simulink model "nms_model"  (Simulink 7.5)
settings: Solver=ode15s  StartTime=0.0  StopTime=60  FixedStep=1e-3  MaxStep=ts_max  RelTol=1e-3  AbsTol=1e-4
InitFcn:
  | nms_model_MechInit
  | nms_model_ControlInit
values from neighbouring files (symbols this model uses):
  c = 0.05    [muscleParams.m]    (also in nms_model_MechInit.m)
  c_jointstop = 0.3 / (pi/180)    (= 17.1887338539)    [muscleParams.m]    (also in nms_model_MechInit.m)
  D12_F = 0.16    [nms_model_MechInit.m]
  D12_S = L_S    (= 0.5)    [nms_model_MechInit.m]
  D12_T = L_T    (= 0.5)    [nms_model_MechInit.m]
  D13_F = 0.20    (= 0.2)    [nms_model_MechInit.m]
  D1G_F = 0.14    [nms_model_MechInit.m]
  D1G_HAT = 0.35    [nms_model_MechInit.m]
  D1G_S = 0.3    [nms_model_MechInit.m]
  D1G_T = 0.3    [nms_model_MechInit.m]
  DeltaThRef = 5e-3    (= 0.005)    [nms_model_MechInit.m]
  eref = 0.04    [muscleParams.m]    (also in nms_model_MechInit.m)
  FmaxGAS = 1500    [nms_model_MechInit.m]
  FmaxGLU = 1500    [nms_model_MechInit.m]
  FmaxHAM = 3000    [nms_model_MechInit.m]
  FmaxHFL = 2000    [nms_model_MechInit.m]
  FmaxSOL = 4000    [nms_model_MechInit.m]
  FmaxTA = 800    [nms_model_MechInit.m]
  FmaxVAS = 300    [muscleParams.m]    (also in nms_model_MechInit.m = 6000)
  GainDeltaTheta = 2 /100*180/pi    (= 1.14591559026)    [nms_model_ControlInit.m]
  GainGAS = 1.1/FmaxGAS    [nms_model_ControlInit.m]
  GainGLU = 0.5/FmaxGLU    [nms_model_ControlInit.m]
  GainHAM = 0.65/FmaxHAM    [nms_model_ControlInit.m]
  GainHAMHFL = 4    [nms_model_ControlInit.m]
  GainHFL = 0.5    [nms_model_ControlInit.m]
  GainKneOverExt = 2    [nms_model_ControlInit.m]
  GainSOL = 1.2/FmaxSOL    [nms_model_ControlInit.m]
  GainSOLTA = 0.4/FmaxSOL    [nms_model_ControlInit.m]
  GainTA = 1.1    [nms_model_ControlInit.m]
  GainVAS = 1.2/FmaxVAS    [nms_model_ControlInit.m]
  In_F = 0.005    [nms_model_MechInit.m]
  In_HAT = 3    [nms_model_MechInit.m]
  In_S = 0.05    [nms_model_MechInit.m]
  In_T = 0.15    [nms_model_MechInit.m]
  K = 5    [muscleParams.m]    (also in nms_model_MechInit.m)
  k_gx = (2*(m_F+m_S+m_T)+m_HAT)*g/0.1    (= 7848)    [nms_model_MechInit.m]
  k_gy = (2*(m_F+m_S+m_T)+m_HAT)*g/0.01    (= 78480)    [nms_model_MechInit.m]
  k_pressure = m_HAT * 9.81 / DeltaThRef    (= 104967)    [nms_model_MechInit.m]
  K_swing = 0.25    [nms_model_ControlInit.m]
  KneePh23Offset = 170*pi/180    (= 2.96705972839)    [nms_model_ControlInit.m]
  LceOffsetHAM = 0.85    [nms_model_ControlInit.m]
  LceOffsetHFL = 0.65    [nms_model_ControlInit.m]
  LceOffsetTA = 1-0.5*w    [nms_model_ControlInit.m]
  LongDelay = 0.020    (= 0.02)    [nms_model_ControlInit.m]
  loptGAS = 0.05    [nms_model_MechInit.m]
  loptGLU = 0.11    [nms_model_MechInit.m]
  loptHAM = 0.10    (= 0.1)    [nms_model_MechInit.m]
  loptHFL = 0.11    [nms_model_MechInit.m]
  loptSOL = 0.04    [nms_model_MechInit.m]
  loptTA = 0.06    [nms_model_MechInit.m]
  loptVAS = 0.13    [muscleParams.m]    (also in nms_model_MechInit.m = 0.08)
  lslackGAS = 0.40    (= 0.4)    [nms_model_MechInit.m]
  lslackGLU = 0.13    [nms_model_MechInit.m]
  lslackHAM = 0.31    [nms_model_MechInit.m]
  lslackHFL = 0.10    (= 0.1)    [nms_model_MechInit.m]
  lslackSOL = 0.26    [nms_model_MechInit.m]
  lslackTA = 0.24    [nms_model_MechInit.m]
  lslackVAS = 0.23    [muscleParams.m]    (also in nms_model_MechInit.m)
  m_F = 1.25    [nms_model_MechInit.m]
  m_HAT = 53.5    [nms_model_MechInit.m]
  m_S = 3.5    [nms_model_MechInit.m]
  m_T = 8.5    [nms_model_MechInit.m]
  MidDelay = 0.010    (= 0.01)    [nms_model_ControlInit.m]
  mu_slide = 0.8    [nms_model_MechInit.m]
  mu_stick = 0.9    [nms_model_MechInit.m]
  N = 1.5    [muscleParams.m]    (also in nms_model_MechInit.m)
  phi12_LowLimit = 70*pi/180    (= 1.2217304764)    [nms_model_MechInit.m]
  phi12_UpLimit = 180*pi/180    (= 3.14159265359)    [muscleParams.m]    (also in nms_model_MechInit.m = 2.26892802759)
  phi23_UpLimit = 159*pi/180    (= 2.77507351067)    [muscleParams.m]    (also in nms_model_MechInit.m = 3.05432619099)
  phi34_UpLimit = 230*pi/180    (= 4.01425727959)    [nms_model_MechInit.m]
  phimaxGASa = 110*pi/180    (= 1.91986217719)    [nms_model_MechInit.m]
  phimaxGASk = 140*pi/180    (= 2.44346095279)    [nms_model_MechInit.m]
  phimaxHAMk = 180*pi/180    (= 3.14159265359)    [nms_model_MechInit.m]
  phimaxSOL = 110*pi/180    (= 1.91986217719)    [nms_model_MechInit.m]
  phimaxTA = 80*pi/180    (= 1.3962634016)    [nms_model_MechInit.m]
  phimaxVAS = 90*pi/180    (= 1.57079632679)    [muscleParams.m]    (also in nms_model_MechInit.m = 2.87979326579)
  phirefGASa = 80*pi/180    (= 1.3962634016)    [nms_model_MechInit.m]
  phirefGASk = 165*pi/180    (= 2.87979326579)    [nms_model_MechInit.m]
  phirefGLU = 150*pi/180    (= 2.61799387799)    [nms_model_MechInit.m]
  phirefHAMh = 155*pi/180    (= 2.70526034059)    [nms_model_MechInit.m]
  phirefHAMk = 180*pi/180    (= 3.14159265359)    [nms_model_MechInit.m]
  phirefHFL = 180*pi/180    (= 3.14159265359)    [nms_model_MechInit.m]
  phirefSOL = 80*pi/180    (= 1.3962634016)    [nms_model_MechInit.m]
  phirefTA = 110*pi/180    (= 1.91986217719)    [nms_model_MechInit.m]
  phirefVAS = 60*pi/180    (= 1.0471975512)    [muscleParams.m]    (also in nms_model_MechInit.m = 2.18166156499)
  PosGainGG = 1/(30*pi/180)    (= 1.9098593171)    [nms_model_ControlInit.m]
  PreStimGAS = 0.01    [nms_model_ControlInit.m]
  PreStimGG = 0.05    [nms_model_ControlInit.m]
  PreStimGLU = 0.01    [nms_model_ControlInit.m]
  PreStimHAM = 0.01    [nms_model_ControlInit.m]
  PreStimHFL = 0.01    [nms_model_ControlInit.m]
  PreStimSOL = 0.01    [nms_model_ControlInit.m]
  PreStimTA = 0.01    [nms_model_ControlInit.m]
  PreStimVAS = 0.08    [nms_model_ControlInit.m]
  rGASa = 0.05    [nms_model_MechInit.m]
  rGASk = 0.05    [nms_model_MechInit.m]
  rGLU = 0.10    (= 0.1)    [nms_model_MechInit.m]
  rHAMh = 0.08    [nms_model_MechInit.m]
  rHAMk = 0.05    [nms_model_MechInit.m]
  rHFL = 0.10    (= 0.1)    [nms_model_MechInit.m]
  rhoGASa = 0.7    [nms_model_MechInit.m]
  rhoGASk = 0.7    [nms_model_MechInit.m]
  rhoGLU = 0.5    [nms_model_MechInit.m]
  rhoHAMh = 0.7    [nms_model_MechInit.m]
  rhoHAMk = 0.7    [nms_model_MechInit.m]
  rhoHFL = 0.5    [nms_model_MechInit.m]
  rhoSOL = 0.5    [nms_model_MechInit.m]
  rhoTA = 0.7    [nms_model_MechInit.m]
  rhoVAS = 3    [muscleParams.m]    (also in nms_model_MechInit.m = 0.7)
  rSOL = 0.05    [nms_model_MechInit.m]
  rTA = 0.04    [nms_model_MechInit.m]
  rVAS = 0.03    [muscleParams.m]    (also in nms_model_MechInit.m = 0.06)
  s = orProblemSendCommand(['LoadIKFastSolver robot Translation3D'],probid)    [init.m]
  ShortDelay = 0.005    [nms_model_ControlInit.m]
  SpeedGainGG = 0.2    [nms_model_ControlInit.m]
  tau = 0.01    [muscleParams.m]    (also in nms_model_MechInit.m)
  Theta0 = 6*pi/180    (= 0.10471975512)    [nms_model_ControlInit.m]
  ThPos = 4/5    (= 0.8)    [nms_model_MechInit.m]
  v_gx_max = 0.03    [nms_model_MechInit.m]
  v_gy_max = 0.03    [nms_model_MechInit.m]
  ... (+11 more)
undefined symbols (not defined in the file or in its folder): sgn
libraries: mblibv1 x60, simulink x22, simulink_extras x20
(part 2 of 9)

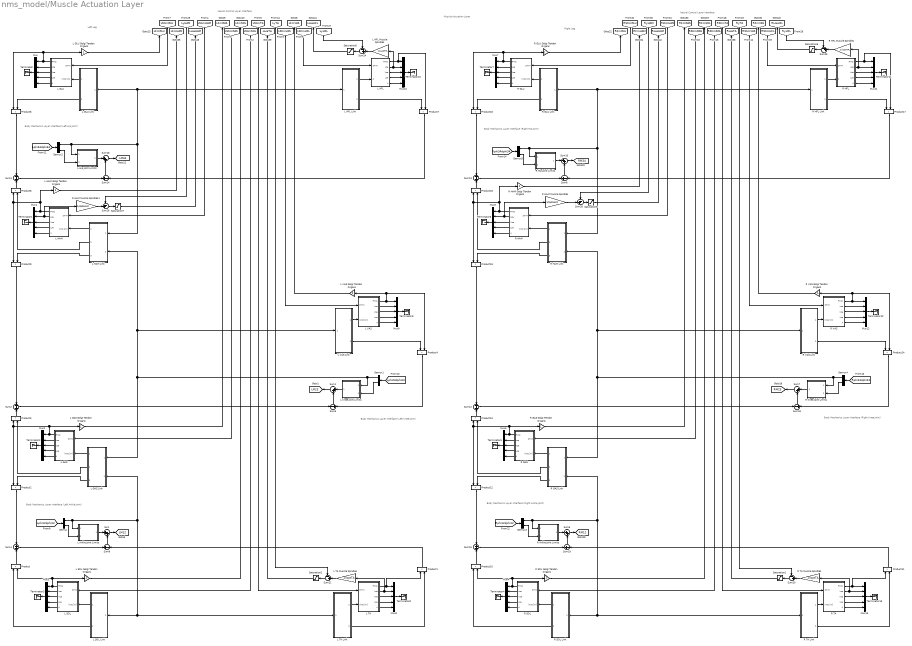
== system nms_model/Muscle Actuation Layer ==
  note: Left Leg
  note: Neural Control Layer Interface
  note: Body Mechanics Layer
      | Interface (Left Hip Joint)
  note: Body Mechanics Layer
      | Interface (Left Knee Joint)
  note: Body Mechanics Layer
      | Interface (Left Ankle Joint)
  note: Neural Control Layer Interface
  note: Body Mechanics Layer
      | Interface (Right Hip Joint)
  note: Body Mechanics Layer
      | Interface (Right Knee Joint)
  note: Body Mechanics Layer
      | Interface (Right Ankle Joint)
  note: Right Leg
  note: Muscle Actuation Layer
  Demux{,1..5} (6 alike) : Demux  Outputs=2
  L Ankle Joint Limits : Subsystem
  L GAS : Subsystem
  L GAS Golgi Tendon Organs : Gain  ParameterDataType=sfix(16)  ParameterScaling=2^0  OutDataType=sfix(16)  OutScaling=2^0
  L GAS Link : Subsystem
  L GLU : Subsystem
  L GLU Golgi Tendon Organs : Gain  ParameterDataType=sfix(16)  ParameterScaling=2^0  OutDataType=sfix(16)  OutScaling=2^0
  L GLU Link : Subsystem
  L HAM : Subsystem
  L HAM Golgi Tendon Organs : Gain  ParameterDataType=sfix(16)  ParameterScaling=2^0  OutDataType=sfix(16)  OutScaling=2^0
  L HAM Link : Subsystem
  L HFL : Subsystem
  L HFL Muscle Spindles : Gain  Gain=1/loptHFL  ParameterDataType=sfix(16)  ParameterScaling=2^0  OutDataType=sfix(16)  OutScaling=2^0
  L HFL Link : Subsystem
  L Hip Joint Limits : Subsystem
  L Knee Joint Limits : Subsystem
  L SOL : Subsystem
  L SOL Golgi Tendon Organs : Gain  ParameterDataType=sfix(16)  ParameterScaling=2^0  OutDataType=sfix(16)  OutScaling=2^0
  L SOL Link : Subsystem
  L TA : Subsystem
  L TA Muscle Spindles : Gain  Gain=1/loptTA  ParameterDataType=sfix(16)  ParameterScaling=2^0  OutDataType=sfix(16)  OutScaling=2^0
  L TA Link : Subsystem
  L VAS : Subsystem
  L VAS Golgi Tendon Organs : Gain  ParameterDataType=sfix(16)  ParameterScaling=2^0  OutDataType=sfix(16)  OutScaling=2^0
  L VAS Link : Subsystem
  Mux{,1..13} (14 alike) : Mux  Inputs=5
  Product{,1..4,6..14,16..19} (18 alike) : Product  OutDataType=sfix(16)  OutScaling=2^0  RndMeth=Zero
  R Ankle Joint Limits : Subsystem
  R GAS : Subsystem
  R GAS Golgi Tendon Organs : Gain  ParameterDataType=sfix(16)  ParameterScaling=2^0  OutDataType=sfix(16)  OutScaling=2^0
  R GAS Link : Subsystem
  R GLU : Subsystem
  R GLU Golgi Tendon Organs : Gain  ParameterDataType=sfix(16)  ParameterScaling=2^0  OutDataType=sfix(16)  OutScaling=2^0
  R GLU Link : Subsystem
  R HAM : Subsystem
  R HAM Golgi Tendon Organs : Gain  ParameterDataType=sfix(16)  ParameterScaling=2^0  OutDataType=sfix(16)  OutScaling=2^0
  R HAM Muscle Spindles : Gain  Gain=1/loptHAM  ParameterDataType=sfix(16)  ParameterScaling=2^0  OutDataType=sfix(16)  OutScaling=2^0
  R HAM Muscle Spindles1 : Gain  Gain=1/loptHAM  ParameterDataType=sfix(16)  ParameterScaling=2^0  OutDataType=sfix(16)  OutScaling=2^0
  R HAM Link : Subsystem
  R HFL : Subsystem
  R HFL Muscle Spindles : Gain  Gain=1/loptHFL  ParameterDataType=sfix(16)  ParameterScaling=2^0  OutDataType=sfix(16)  OutScaling=2^0
  R HFL Link : Subsystem
  R Hip Joint Limits : Subsystem
  R Knee Joint Limits : Subsystem
  R SOL : Subsystem
  R SOL Golgi Tendon Organs : Gain  ParameterDataType=sfix(16)  ParameterScaling=2^0  OutDataType=sfix(16)  OutScaling=2^0
  R SOL Link : Subsystem
  R TA : Subsystem
  R TA Muscle Spindles : Gain  Gain=1/loptTA  ParameterDataType=sfix(16)  ParameterScaling=2^0  OutDataType=sfix(16)  OutScaling=2^0
  R TA Link : Subsystem
  R VAS : Subsystem
  R VAS Golgi Tendon Organs : Gain  ParameterDataType=sfix(16)  ParameterScaling=2^0  OutDataType=sfix(16)  OutScaling=2^0
  R VAS Link : Subsystem
  Saturation{1..2,5..7,9} (6 alike) : Saturate  UpperLimit=inf  LowerLimit=0  ZeroCross=off
  Sum{,1,6..7,10,16} (6 alike) : Sum  Inputs=|++  OutDataType=sfix(16)  OutScaling=2^0
  Sum{2..4,12..13,15} (6 alike) : Sum  OutDataType=sfix(16)  OutScaling=2^0
  Sum{8..9,14,19} (4 alike) : Sum  Inputs=+-  OutDataType=sfix(16)  OutScaling=2^0
  Sum18 : Sum  Inputs=-+  OutDataType=sfix(16)  OutScaling=2^0
  Sum{20..21,24..26,28} (6 alike) : Sum  Inputs=-+|  OutDataType=sfix(16)  OutScaling=2^0  SaturateOnIntegerOverflow=on  InputSameDT=on  OutDataTypeStr=Inherit: Same as first input
  Sum5 : Sum  Inputs=-+  OutDataType=sfix(16)  OutScaling=2^0
  Terminator{,1..13} (14 alike) : Terminator
  tag scope: LFmGAS=global, LFmGLU=global, LFmHAM=global, LFmSOL=global, LFmVAS=global, LLceHAM=global, LLceHFL=global, LLceTA=global, LM12=global, LM23=global, LM34=global, RFmGAS=global, RFmGLU=global, RFmHAM=global, RFmSOL=global, RFmVAS=global, RLceHAM=global, RLceHFL=global, RLceTA=global, RM12=global, RM23=global, RM34=global
  wires:
  Demux1/1 -> L Knee Joint Limits/1(phi [rad]), L VAS Link/1(phi23 [rad]), L HAM Link/2(phi23 [rad]), L GAS Link/1(phi23 [rad])
  L SOL/1(Fmtc) -> Product/2, L SOL Golgi Tendon Organs/1, Mux3/1
  L TA/1(Fmtc) -> Product1/1, Mux8/1
  L TA/2(Lce) -> L TA Muscle Spindles/1, Mux8/2
  L TA/5(A) -> Mux8/5
  L GAS/1(Fmtc) -> Product2/1, Product3/1, L GAS Golgi Tendon Organs/1, Mux2/1
  Demux/1 -> L SOL Link/1(phi12 [rad]), L TA Link/1(phi12 [rad]), L GAS Link/2(phi12 [rad]), L Ankle Joint Limits/1(phi [rad])
  [LStimTA] -> L TA/1(STIM)
  [LStimSOL] -> L SOL/1(STIM)
  [LStimHAM] -> L HAM/1(STIM)
  L HAM/1(Fmtc) -> Product9/1, Product8/1, L HAM Golgi Tendon Organs/1, Mux1/1
  L HAM/2(Lce) -> R HAM Muscle Spindles1/1, Mux1/2
  L HFL/1(Fmtc) -> Product7/2, Mux10/1
  L HFL/2(Lce) -> L HFL Muscle Spindles/1, Mux10/2
  [LStimHFL] -> L HFL/1(STIM)
  L GLU/1(Fmtc) -> Product6/1, L GLU Golgi Tendon Organs/1, Mux/1
  [LStimGLU] -> L GLU/1(STIM)
  Sum16/1 -> [LM34]
  Demux/2 -> L Ankle Joint Limits/2(dphi [rad/s])
  Sum9/1 -> Sum/2
  Demux1/2 -> L Knee Joint Limits/2(dphi [rad/s])
  L SOL Link/1(lmtc [m]) -> L SOL/2(lmtc [m])
  L TA Link/1(lmtc [m]) -> L TA/2(lmtc [m])
  L GAS Link/3(lever12 [m]) -> Product2/2
  L GAS Link/2(lever23 [m]) -> Product3/2
  [LStimGAS] -> L GAS/1(STIM)
  L GAS Link/1(lmtu [m]) -> L GAS/2(lmtc [m])
  L VAS Link/1(lmtu [m]) -> L VAS/2(lmtc [m])
  Product4/1 -> Sum5/2
  L HAM Link/1(lmtu [m]) -> L HAM/2(lmtc [m])
  L HAM Link/2(lever34 [m]) -> Product8/2
  L HAM Link/3(lever23 [m]) -> Product9/2
  Product9/1 -> Sum2/1
  Product3/1 -> Sum2/2
  Sum3/1 -> Sum14/1
  Sum4/1 -> Sum9/1
  [Lphi12dphi12] -> Demux/1
  [Lphi23dphi23] -> Demux1/1
  [Lphi34dphi34] -> Demux2/1
  Demux2/1 -> L Hip Joint Limits/1(phi [rad]), L HFL Link/1(phi34 [rad]), L GLU Link/1(phi34 [rad]), L HAM Link/1(phi34 [rad])
  L SOL Link/2(lever [m]) -> Product/1
  Product/1 -> Sum4/2
  Product2/1 -> Sum4/1
  L TA Link/2(lever [m]) -> Product1/2
  Product1/1 -> Sum9/2
  L Ankle Joint Limits/1(M_stop [Nm]) -> Sum/1
  Sum/1 -> [LM12]
  L SOL/5(A) -> Mux3/5
  L GAS/5(A) -> Mux2/5
  L VAS/5(A) -> Mux9/5
  L VAS/1(Fmtc) -> Product4/2, L VAS Golgi Tendon Organs/1, Mux9/1
  Sum1/1 -> [LM23]
  L Knee Joint Limits/1(M_stop [Nm]) -> Sum1/1
  Sum5/1 -> Sum1/2
  L VAS Link/2(lever [m]) -> Product4/1
  Sum2/1 -> Sum5/1
  L HAM/5(A) -> Mux1/5
  Product8/1 -> Sum3/2
  Product6/1 -> Sum3/1
  L GLU Link/1(lmtu [m]) -> L GLU/2(lmtc [m])
  L GLU Link/2(lever [m]) -> Product6/2
  L GLU/5(A) -> Mux/5
  Demux2/2 -> L Hip Joint Limits/2(dphi [rad/s])
  L Hip Joint Limits/1(M_stop [Nm]) -> Sum16/1
  Sum14/1 -> Sum16/2
  Product7/1 -> Sum14/2
  L HFL Link/1(lmtu [m]) -> L HFL/2(lmtc [m])
  L HFL/5(A) -> Mux10/5
  L HFL Link/2(lever [m]) -> Product7/1
  [LStimVAS] -> L VAS/1(STIM)
  L SOL Golgi Tendon Organs/1 -> [LFmSOL]
  L GAS Golgi Tendon Organs/1 -> [LFmGAS]
  L VAS Golgi Tendon Organs/1 -> [LFmVAS]
  Demux4/1 -> R Knee Joint Limits/1(phi [rad]), R VAS Link/1(phi23 [rad]), R HAM Link/2(phi23 [rad]), R GAS Link/1(phi23 [rad])
  R SOL/1(Fmtc) -> Product10/2, R SOL Golgi Tendon Organs/1, Mux4/1
  R TA/1(Fmtc) -> Product11/1, Mux13/1
  R TA/2(Lce) -> R TA Muscle Spindles/1, Mux13/2
  R TA/5(A) -> Mux13/5
  R GAS/1(Fmtc) -> Product12/1, Product13/1, R GAS Golgi Tendon Organs/1, Mux5/1
  Demux3/1 -> R SOL Link/1(phi12 [rad]), R TA Link/1(phi12 [rad]), R GAS Link/2(phi12 [rad]), R Ankle Joint Limits/1(phi [rad])
  [RStimTA] -> R TA/1(STIM)
  [RStimSOL] -> R SOL/1(STIM)
  R HAM/1(Fmtc) -> Product19/1, Product18/1, R HAM Golgi Tendon Organs/1, Mux6/1
  R HAM/2(Lce) -> R HAM Muscle Spindles/1, Mux6/2
  R HFL/1(Fmtc) -> Product17/2, Mux11/1
  R HFL/2(Lce) -> R HFL Muscle Spindles/1, Mux11/2
  [RStimHFL] -> R HFL/1(STIM)
  R GLU/1(Fmtc) -> Product16/1, R GLU Golgi Tendon Organs/1, Mux7/1
  Sum10/1 -> [RM34]
  Demux3/2 -> R Ankle Joint Limits/2(dphi [rad/s])
  Sum19/1 -> Sum6/2
  Demux4/2 -> R Knee Joint Limits/2(dphi [rad/s])
  R SOL Link/1(lmtc [m]) -> R SOL/2(lmtc [m])
  R GAS Link/3(lever12 [m]) -> Product12/2
  R GAS Link/2(lever23 [m]) -> Product13/2
  [RStimGAS] -> R GAS/1(STIM)
  R GAS Link/1(lmtu [m]) -> R GAS/2(lmtc [m])
  R VAS Link/1(lmtu [m]) -> R VAS/2(lmtc [m])
  Product14/1 -> Sum18/2
  R HAM Link/1(lmtu [m]) -> R HAM/2(lmtc [m])
  R HAM Link/2(lever34 [m]) -> Product18/2
  R HAM Link/3(lever23 [m]) -> Product19/2
  Product19/1 -> Sum12/1
  Product13/1 -> Sum12/2
  Sum13/1 -> Sum8/1
  Sum15/1 -> Sum19/1
  [Rphi12dphi12] -> Demux3/1
  [Rphi23dphi23] -> Demux4/1
  [Rphi34dphi34] -> Demux5/1
  Demux5/1 -> R Hip Joint Limits/1(phi [rad]), R HFL Link/1(phi34 [rad]), R GLU Link/1(phi34 [rad]), R HAM Link/1(phi34 [rad])
  R SOL Link/2(lever [m]) -> Product10/1
  Product10/1 -> Sum15/2
  Product12/1 -> Sum15/1
  R TA Link/2(lever [m]) -> Product11/2
  Product11/1 -> Sum19/2
  R Ankle Joint Limits/1(M_stop [Nm]) -> Sum6/1
  Sum6/1 -> [RM12]
  R SOL/5(A) -> Mux4/5
  R GAS/5(A) -> Mux5/5
  R VAS/5(A) -> Mux12/5
  R VAS/1(Fmtc) -> Product14/2, R VAS Golgi Tendon Organs/1, Mux12/1
  Sum7/1 -> [RM23]
  R Knee Joint Limits/1(M_stop [Nm]) -> Sum7/1
  Sum18/1 -> Sum7/2
  R VAS Link/2(lever [m]) -> Product14/1
  Sum12/1 -> Sum18/1
  R HAM/5(A) -> Mux6/5
  Product18/1 -> Sum13/2
  Product16/1 -> Sum13/1
  R GLU Link/1(lmtu [m]) -> R GLU/2(lmtc [m])
  R GLU Link/2(lever [m]) -> Product16/2
  R GLU/5(A) -> Mux7/5
  Demux5/2 -> R Hip Joint Limits/2(dphi [rad/s])
  R Hip Joint Limits/1(M_stop [Nm]) -> Sum10/1
  Sum8/1 -> Sum10/2
  Product17/1 -> Sum8/2
  R HFL Link/1(lmtu [m]) -> R HFL/2(lmtc [m])
  R HFL/5(A) -> Mux11/5
  R HFL Link/2(lever [m]) -> Product17/1
  [RStimVAS] -> R VAS/1(STIM)
  R SOL Golgi Tendon Organs/1 -> [RFmSOL]
  R GAS Golgi Tendon Organs/1 -> [RFmGAS]
  R VAS Golgi Tendon Organs/1 -> [RFmVAS]
  R HAM Golgi Tendon Organs/1 -> [RFmHAM]
  L HAM Golgi Tendon Organs/1 -> [LFmHAM]
  R TA Muscle Spindles/1 -> Sum20/2
  Sum20/1 -> Saturation1/1
  [RyTA] -> Sum20/1
  Saturation1/1 -> [RLceTA]
  L TA Muscle Spindles/1 -> Sum21/2
  Sum21/1 -> Saturation2/1
  [LyTA] -> Sum21/1
  Saturation2/1 -> [LLceTA]
  L HFL Muscle Spindles/1 -> Sum24/2
  Sum24/1 -> Saturation5/1
  [LyHFL] -> Sum24/1
  R HFL Muscle Spindles/1 -> Sum25/2
  Sum25/1 -> Saturation6/1
  [RyHFL] -> Sum25/1
  Saturation5/1 -> [LLceHFL]
  Saturation6/1 -> [RLceHFL]
  R HAM Muscle Spindles/1 -> Sum28/2
  Sum28/1 -> Saturation9/1
  Saturation9/1 -> [RLceHAM]
  R HAM Muscle Spindles1/1 -> Sum26/2
  Sum26/1 -> Saturation7/1
  [LyHAM] -> Sum26/1
  Saturation7/1 -> [LLceHAM]
  [RStimHAM] -> R HAM/1(STIM)
  [RStimGLU] -> R GLU/1(STIM)
  [RyHAM] -> Sum28/1
  R TA Link/1(lmtc [m]) -> R TA/2(lmtc [m])
  L GLU Golgi Tendon Organs/1 -> [LFmGLU]
  R GLU Golgi Tendon Organs/1 -> [RFmGLU]
  L GLU/2(Lce) -> Mux/2
  L GLU/3(Vce) -> Mux/3
  L GLU/4(Lse) -> Mux/4
  Mux/1 -> Terminator/1
  Mux1/1 -> Terminator1/1
  L HAM/4(Lse) -> Mux1/4
  L HAM/3(Vce) -> Mux1/3
  Mux2/1 -> Terminator2/1
  L GAS/4(Lse) -> Mux2/4
  L GAS/3(Vce) -> Mux2/3
  L GAS/2(Lce) -> Mux2/2
  Mux3/1 -> Terminator3/1
  L SOL/2(Lce) -> Mux3/2
  L SOL/3(Vce) -> Mux3/3
  L SOL/4(Lse) -> Mux3/4
  Mux4/1 -> Terminator4/1
  R SOL/4(Lse) -> Mux4/4
  R SOL/3(Vce) -> Mux4/3
  R SOL/2(Lce) -> Mux4/2
  Mux5/1 -> Terminator5/1
  R GAS/4(Lse) -> Mux5/4
  R GAS/3(Vce) -> Mux5/3
  R GAS/2(Lce) -> Mux5/2
  Mux6/1 -> Terminator6/1
  R HAM/3(Vce) -> Mux6/3
  R HAM/4(Lse) -> Mux6/4
  Mux7/1 -> Terminator7/1
  R GLU/2(Lce) -> Mux7/2
  R GLU/3(Vce) -> Mux7/3
  R GLU/4(Lse) -> Mux7/4
  Mux8/1 -> Terminator8/1
  L TA/4(Lse) -> Mux8/4
  L TA/3(Vce) -> Mux8/3
  Mux9/1 -> Terminator9/1
  L VAS/4(Lse) -> Mux9/4
  L VAS/3(Vce) -> Mux9/3
  L VAS/2(Lce) -> Mux9/2
  Mux10/1 -> Terminator10/1
  L HFL/4(Lse) -> Mux10/4
  L HFL/3(Vce) -> Mux10/3
  Mux11/1 -> Terminator11/1
  R HFL/4(Lse) -> Mux11/4
  R HFL/3(Vce) -> Mux11/3
  Mux12/1 -> Terminator12/1
  R VAS/2(Lce) -> Mux12/2
  R VAS/3(Vce) -> Mux12/3
  R VAS/4(Lse) -> Mux12/4
  Mux13/1 -> Terminator13/1
  R TA/3(Vce) -> Mux13/3
  R TA/4(Lse) -> Mux13/4

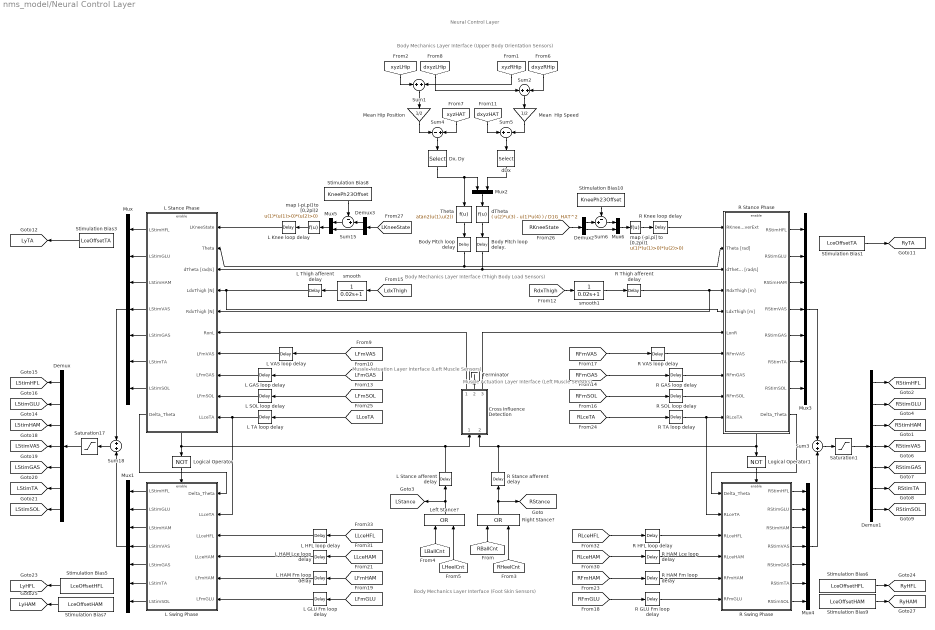
== system nms_model/Neural Control Layer ==
  note: Body Mechanics Layer Interface
      | (Foot Skin Sensors)
  note: Neural Control Layer
  note: Body Mechanics Layer Interface
      | (Upper Body Orientation Sensors)
  note: Body Mechanics Layer Interface
      | (Thigh Body Load Sensors)
  note: Muscle
      | Actuation
      | Layer
      | Interface
      | (Left
      | Muscle
      | Sensors)
  note: Muscle
      | Actuation
      | Layer
      | Interface
      | (Left
      | Muscle
      | Sensors)
  " Mean  Hip Speed" : Gain  Gain=1/2  ParameterDataType=sfix(16)  ParameterScaling=2^0  OutDataType=sfix(16)  OutScaling=2^0
  Body Pitch loop delay : TransportDelay  DelayTime=ShortDelay
  Body Pitch loop delay. : TransportDelay  DelayTime=ShortDelay
  Cross Influence Detection : Subsystem
  Demux : Demux  Outputs=7
  Demux1 : Demux  Outputs=7
  Demux2 : Demux  Outputs=2
  Demux3 : Demux  Outputs=2
  "Dx, Dy" : Selector  InputPortWidth=3  IndexOptions=Index vector (dialog)  Indices=[1 2]  OutputSizes=1
  L GAS loop delay : TransportDelay  DelayTime=LongDelay
  L GLU Fm loop delay : TransportDelay  DelayTime=ShortDelay
  L HAM Fm loop delay : TransportDelay  DelayTime=ShortDelay
  L HAM Lce loop delay : TransportDelay  DelayTime=ShortDelay
  L HFL loop delay : TransportDelay  DelayTime=ShortDelay
  L Knee loop delay : TransportDelay  DelayTime=MidDelay
  L SOL loop delay : TransportDelay  DelayTime=LongDelay
  L Stance afferent delay : TransportDelay  DelayTime=MidDelay
  L Stance Phase : Subsystem  TreatAsAtomicUnit=on
  L Swing Phase : Subsystem  TreatAsAtomicUnit=on
  L TA loop delay : TransportDelay  DelayTime=LongDelay
  L Thigh afferent delay : TransportDelay  DelayTime=ShortDelay
  L VAS loop delay : TransportDelay  DelayTime=MidDelay
  Left Stance? : Logic  Operator=OR  AllPortsSameDT=off
  Logical Operator : Logic  Operator=NOT  AllPortsSameDT=off  OutDataTypeMode=boolean  OutDataTypeStr=boolean
  Logical Operator1 : Logic  Operator=NOT  AllPortsSameDT=off  OutDataTypeMode=boolean  OutDataTypeStr=boolean
  Mean Hip Position : Gain  Gain=1/2  ParameterDataType=sfix(16)  ParameterScaling=2^0  OutDataType=sfix(16)  OutScaling=2^0
  Mux{,1,3..4} (4 alike) : Mux  Inputs=7
  Mux2 : Mux  Inputs=2
  Mux5 : Mux  Inputs=2
  Mux6 : Mux  Inputs=2
  R GAS loop delay : TransportDelay  DelayTime=LongDelay
  R GLU Fm loop delay : TransportDelay  DelayTime=ShortDelay
  R HAM Fm loop delay : TransportDelay  DelayTime=ShortDelay
  R HAM Lce loop delay : TransportDelay  DelayTime=ShortDelay
  R HFL loop delay : TransportDelay  DelayTime=ShortDelay
  R Knee loop delay : TransportDelay  DelayTime=MidDelay
  R SOL loop delay : TransportDelay  DelayTime=LongDelay
  R Stance afferent delay : TransportDelay  DelayTime=MidDelay
  R Stance Phase : Subsystem  TreatAsAtomicUnit=on
  R Swing Phase : Subsystem  TreatAsAtomicUnit=on
  R TA loop delay : TransportDelay  DelayTime=LongDelay
  R Thigh afferent delay : TransportDelay  DelayTime=ShortDelay
  R VAS loop delay : TransportDelay  DelayTime=MidDelay
  Right Stance? : Logic  Operator=OR  AllPortsSameDT=off
  Saturation1 : Saturate  UpperLimit=1  LowerLimit=0.01
  Saturation17 : Saturate  UpperLimit=1  LowerLimit=0.01  ZeroCross=off
  Stimulation Bias1 : Constant  Value=LceOffsetTA  OutDataType=sfix(16)  OutScaling=2^0
  Stimulation Bias10 : Constant  Value=KneePh23Offset  OutDataType=sfix(16)  OutScaling=2^0
  Stimulation Bias3 : Constant  Value=LceOffsetTA  OutDataType=sfix(16)  OutScaling=2^0
  Stimulation Bias5 : Constant  Value=LceOffsetHFL  OutDataType=sfix(16)  OutScaling=2^0
  Stimulation Bias6 : Constant  Value=LceOffsetHFL  OutDataType=sfix(16)  OutScaling=2^0
  Stimulation Bias7 : Constant  Value=LceOffsetHAM  OutDataType=sfix(16)  OutScaling=2^0
  Stimulation Bias8 : Constant  Value=KneePh23Offset  OutDataType=sfix(16)  OutScaling=2^0
  Stimulation Bias9 : Constant  Value=LceOffsetHAM  OutDataType=sfix(16)  OutScaling=2^0
  Sum{1..3,18} (4 alike) : Sum  OutDataType=sfix(16)  OutScaling=2^0
  Sum15 : Sum  Inputs=-+|  OutDataType=sfix(16)  OutScaling=2^0  SaturateOnIntegerOverflow=on  InputSameDT=on  OutDataTypeStr=Inherit: Same as first input
  Sum4 : Sum  Inputs=-+  OutDataType=sfix(16)  OutScaling=2^0
  Sum5 : Sum  Inputs=+-  OutDataType=sfix(16)  OutScaling=2^0
  Sum6 : Sum  Inputs=-+|  OutDataType=sfix(16)  OutScaling=2^0  SaturateOnIntegerOverflow=on  InputSameDT=on  OutDataTypeStr=Inherit: Same as first input
  Terminator : Terminator
  Theta : Fcn  Expr=atan2(u(1),u(2))
  dDx : Selector  InputPortWidth=3  IndexOptions=Index vector (dialog)  Indices=[1 2]  OutputSizes=1
  dTheta : Fcn  Expr=( u(2)*u(3) - u(1)*u(4) ) / D1G_HAT^2
  map (-pi,pi] to [0,2pi)1 : Fcn  Expr=u(1)*(u(1)>0)*(u(2)>0)
  map (-pi,pi] to [0,2pi)2 : Fcn  Expr=u(1)*(u(1)>0)*(u(2)>0)
  smooth : TransferFcn  Denominator=[0.02 1]
  smooth1 : TransferFcn  Denominator=[0.02 1]
  tag scope: LStance=global, LStimGAS=global, LStimGLU=global, LStimHAM=global, LStimHFL=global, LStimSOL=global, LStimTA=global, LStimVAS=global, LyHAM=global, LyHFL=global, LyTA=global, RStance=global, RStimGAS=global, RStimGLU=global, RStimHAM=global, RStimHFL=global, RStimSOL=global, RStimTA=global, RStimVAS=global, RyHAM=global, RyHFL=global, RyTA=global
  wires:
  [RBallCnt] -> Right Stance?/1
  Right Stance?/1 -> R Stance afferent delay/1, [RStance]
  Left Stance?/1 -> L Stance afferent delay/1, [LStance]
  [LHeelCnt] -> Left Stance?/2
  [LBallCnt] -> Left Stance?/1
  [RHeelCnt] -> Right Stance?/2
  Logical Operator/1 -> L Swing Phase/Enable
  Logical Operator1/1 -> R Swing Phase/Enable
  Sum4/1 -> "Dx, Dy"/1
  [dxyzHAT] -> Sum5/1
  Sum5/1 -> dDx/1
  dDx/1 -> Mux2/2
  Mux2/1 -> dTheta/1
  [xyzLHip] -> Sum1/1
  [xyzRHip] -> Sum1/2
  Sum1/1 -> Mean Hip Position/1
  [dxyzLHip] -> Sum2/1
  [dxyzRHip] -> Sum2/2
  Sum2/1 -> " Mean  Hip Speed"/1
  [xyzHAT] -> Sum4/2
  Mean Hip Position/1 -> Sum4/1
  " Mean  Hip Speed"/1 -> Sum5/2
  Theta/1 -> Body Pitch loop delay/1
  dTheta/1 -> Body Pitch loop delay./1
  [LFmVAS] -> L VAS loop delay/1
  [LFmGAS] -> L GAS loop delay/1
  [LFmSOL] -> L SOL loop delay/1
  L SOL loop delay/1 -> L Stance Phase/9(LFmSOL)
  L GAS loop delay/1 -> L Stance Phase/8(LFmGAS)
  L VAS loop delay/1 -> L Stance Phase/7(LFmVAS)
  Cross Influence Detection/3(LonR) -> R Stance Phase/6(LonR)
  Body Pitch loop delay/1 -> L Stance Phase/2(Theta), R Stance Phase/2(Theta [rad])
  Body Pitch loop delay./1 -> R Stance Phase/3(dTheta [rad/s]), L Stance Phase/3(dTheta [rad/s])
  [RFmSOL] -> R SOL loop delay/1
  [RFmGAS] -> R GAS loop delay/1
  [RFmVAS] -> R VAS loop delay/1
  R VAS loop delay/1 -> R Stance Phase/7(RFmVAS)
  R GAS loop delay/1 -> R Stance Phase/8(RFmGAS)
  R SOL loop delay/1 -> R Stance Phase/9(RFmSOL)
  L Swing Phase/1(LStimHFL) -> Mux1/1
  L Swing Phase/2(LStimGLU) -> Mux1/2
  L Swing Phase/3(LStimHAM) -> Mux1/3
  Mux/1 -> Sum18/1
  Mux1/1 -> Sum18/2
  Sum18/1 -> Saturation17/1
  Demux/1 -> [LStimHFL]
  Demux/2 -> [LStimGLU]
  Demux/3 -> [LStimHAM]
  Saturation17/1 -> Demux/1
  Mux3/1 -> Sum3/1
  Mux4/1 -> Sum3/2
  Sum3/1 -> Saturation1/1
  Demux1/1 -> [RStimHFL]
  Demux1/2 -> [RStimGLU]
  Demux1/3 -> [RStimHAM]
  Saturation1/1 -> Demux1/1
  R Stance Phase/1(RStimHFL) -> Mux3/1
  R Stance Phase/2(RStimGLU) -> Mux3/2
  R Stance Phase/3(RStimHAM) -> Mux3/3
  R Swing Phase/1(RStimHFL) -> Mux4/1
  [LFmHAM] -> L HAM Fm loop delay/1
  [LdxThigh] -> smooth/1
  [RdxThigh] -> smooth1/1
  R Thigh afferent delay/1 -> L Stance Phase/5(RdxThigh [N]), R Stance Phase/4(RdxThigh [m])
  [RFmHAM] -> R HAM Fm loop delay/1
  R Swing Phase/2(RStimGLU) -> Mux4/2
  R Swing Phase/3(RStimHAM) -> Mux4/3
  R TA loop delay/1 -> R Stance Phase/10(RLceTA), R Swing Phase/2(RLceTA)
  L TA loop delay/1 -> L Swing Phase/2(LLceTA), L Stance Phase/10(LLceTA)
  Stimulation Bias3/1 -> [LyTA]
  Stimulation Bias1/1 -> [RyTA]
  [RKneeState] -> Demux2/1
  Stimulation Bias5/1 -> [LyHFL]
  Stimulation Bias6/1 -> [RyHFL]
  [RLceHAM] -> R HAM Lce loop delay/1
  R HAM Lce loop delay/1 -> R Swing Phase/4(RLceHAM)
  [RLceHFL] -> R HFL loop delay/1
  Stimulation Bias9/1 -> [RyHAM]
  [LLceHAM] -> L HAM Lce loop delay/1
  [LLceHFL] -> L HFL loop delay/1
  L HAM Lce loop delay/1 -> L Swing Phase/4(LLceHAM)
  Stimulation Bias7/1 -> [LyHAM]
  L HAM Fm loop delay/1 -> L Swing Phase/5(LFmHAM)
  R HAM Fm loop delay/1 -> R Swing Phase/5(RFmHAM)
  smooth/1 -> L Thigh afferent delay/1
  smooth1/1 -> R Thigh afferent delay/1
  R Stance Phase/8(Delta_Theta) -> R Swing Phase/1(Delta_Theta)
  L Stance Phase/8(Delta_Theta) -> L Swing Phase/1(Delta_Theta)
  R Stance afferent delay/1 -> Logical Operator1/1, R Stance Phase/Enable, Cross Influence Detection/2(RStance)
  L Stance afferent delay/1 -> Logical Operator/1, L Stance Phase/Enable, Cross Influence Detection/1(LStance)
  L Thigh afferent delay/1 -> L Stance Phase/4(LdxThigh [N]), R Stance Phase/5(LdxThigh [m])
  Demux3/1 -> Sum15/2
  Demux3/2 -> Mux5/2
  Sum15/1 -> Mux5/1
  Mux5/1 -> map (-pi,pi] to [0,2pi)2/1
  map (-pi,pi] to [0,2pi)2/1 -> L Knee loop delay/1
  Stimulation Bias8/1 -> Sum15/1
  Demux2/1 -> Sum6/2
  Demux2/2 -> Mux6/2
  Sum6/1 -> Mux6/1
  Mux6/1 -> map (-pi,pi] to [0,2pi)1/1
  map (-pi,pi] to [0,2pi)1/1 -> R Knee loop delay/1
  Stimulation Bias10/1 -> Sum6/1
  L Knee loop delay/1 -> L Stance Phase/1(LKneeState)
  [LKneeState] -> Demux3/1
  R Knee loop delay/1 -> R Stance Phase/1(RKneeOverExt)
  Cross Influence Detection/1(RonL) -> L Stance Phase/6(RonL)
  Cross Influence Detection/2(Flight) -> Terminator/1
  [LLceTA] -> L TA loop delay/1
  [RLceTA] -> R TA loop delay/1
  "Dx, Dy"/1 -> Mux2/1, Theta/1
  L Stance Phase/1(LStimHFL) -> Mux/1
  L Stance Phase/2(LStimGLU) -> Mux/2
  L Stance Phase/3(LStimHAM) -> Mux/3
  L Stance Phase/4(LStimVAS) -> Mux/4
  L Stance Phase/5(LStimGAS) -> Mux/5
  L Stance Phase/6(LStimTA) -> Mux/6
  L Stance Phase/7(LStimSOL) -> Mux/7
  Demux/4 -> [LStimVAS]
  Demux/5 -> [LStimGAS]
  Demux/6 -> [LStimTA]
  Demux/7 -> [LStimSOL]
  L Swing Phase/4(LStimVAS) -> Mux1/4
  L Swing Phase/5(LStimGAS) -> Mux1/5
  L Swing Phase/6(LStimTA) -> Mux1/6
  L Swing Phase/7(LStimSOL) -> Mux1/7
  R Stance Phase/4(RStimVAS) -> Mux3/4
  R Stance Phase/5(RStimGAS) -> Mux3/5
  R Stance Phase/6(RStimTA) -> Mux3/6
  R Stance Phase/7(RStimSOL) -> Mux3/7
  R Swing Phase/4(RStimVAS) -> Mux4/4
  R Swing Phase/5(RStimGAS) -> Mux4/5
  R Swing Phase/6(RStimTA) -> Mux4/6
  R Swing Phase/7(RStimSOL) -> Mux4/7
  Demux1/4 -> [RStimVAS]
  Demux1/5 -> [RStimGAS]
  Demux1/6 -> [RStimTA]
  Demux1/7 -> [RStimSOL]
  L HFL loop delay/1 -> L Swing Phase/3(LLceHFL)
  R HFL loop delay/1 -> R Swing Phase/3(RLceHFL)
  [RFmGLU] -> R GLU Fm loop delay/1
  [LFmGLU] -> L GLU Fm loop delay/1
  R GLU Fm loop delay/1 -> R Swing Phase/6(RFmGLU)
  L GLU Fm loop delay/1 -> L Swing Phase/6(LFmGLU)

== system nms_model/Body Mechanics Layer/Left Ball Contact ==
  note: Planar Ground Interaction Model
  Body Actuator : mblibv1/Sensors &  Actuators/Body Actuator  DialogController=MECH.DynMechDlgSource  SystemSampleTime=-1  UpdateFromCAD=off  PhysicalDomain=Mechanical  PortType=blob  ActuationStyle=Force  AngleUnits=deg  ArcVelocityUnits=deg/s  ArcAccelerationUnits=deg/s^2  CoordPositionUnits=m  VelocityUnits=m/s  AccelerationUnits=m/s^2  ForceUnits=N  TorqueUnits=N-m  ActiveIO=on  Width=3  DialogClass=MechanicalActuatorBlock  ReferenceFrame=Absolute (World)  Angle=off  CoordPosition=on  Force=on  Torque=off
  Body Sensor : mblibv1/Sensors &  Actuators/Body Sensor  DialogController=MECH.DynMechDlgSource  SystemSampleTime=-1  UpdateFromCAD=off  PhysicalDomain=Mechanical  PortType=blob  Muxed=on  Pose=off  Angle=on  AngleUnits=deg  ArcVelocity=off  ArcVelocityUnits=deg/s  ArcAcceleration=off  ArcAccelerationUnits=deg/s^2  CoordPosition=on  CoordPositionUnits=m  Velocity=on  VelocityUnits=m/s  Acceleration=off  AccelerationUnits=m/s^2  Quaternion=on  QuaternionDT=off  QuaternionDDT=off  QuaternionUnits=off  OutputVector=[ 3 3 ]  ActiveIO=on  Width=6  DialogClass=MechanicalSensorBlock  ReferenceFrame=Absolute (World)
  Demux1 : Demux
  Ground Friction Model : Subsystem
  Ground1 : Ground
  Mechanical Branching Bar : mblibv1/Utilities/Mechanical Branching Bar  DialogController=MECH.DynMechDlgSource  PhysicalDomain=mechanical  SubClassName=Unknown  LeftPortType=blob  RightPortType=blob  LConnTagsString=_newl0  RConnTagsString=SA0|SA1  UpdateFromCAD=off  DialogClass=MechanicalBranchingBarBlock  NumSAPorts=2
  Mux : Mux  Inputs=2
  Mux1 : Mux  Inputs=3
  Sum : Sum  Inputs=-+|  OutDataType=sfix(16)  OutScaling=2^0
  Terminator : Terminator
  "[y y' x x']" : Selector  InputPortWidth=6  IndexOptions=Index vector (dialog)  Indices=[2 5 1 4]  OutputSizes=1
  contact? : simulink/Logic and Bit Operations/Compare To Zero  SystemSampleTime=-1  relop=<=  LogicOutDataTypeMode=boolean
  yGround : Constant  Value=0  OutDataType=fixdt(1, 16)  OutScaling=2^0
  F : PMIOPort  Port=1  Side=Left
  LBallCnt : Outport  OutDataType=sfix(16)  OutScaling=2^0
  GRF [N N] : Outport  Port=2  OutDataType=sfix(16)  OutScaling=2^0
  wires:
  contact?/1 -> Ground Friction Model/Enable, LBallCnt/1
  Ground Friction Model/1(Fy_Ground[N]) -> Mux/2, Mux1/2
  Ground Friction Model/2(Fx_Friction [N]) -> Mux/1, Mux1/1
  Ground Friction Model/3(Stiction!) -> Terminator/1
  Mux/1 -> GRF [N N]/1
  yGround/1 -> Sum/1
  Sum/1 -> Ground Friction Model/1(dy [m]), contact?/1
  Body Sensor/1 -> "[y y' x x']"/1
  Mux1/1 -> Body Actuator/1
  Demux1/1 -> Sum/2
  Demux1/2 -> Ground Friction Model/2(vy [m/s])
  Demux1/3 -> Ground Friction Model/3(x [m])
  Demux1/4 -> Ground Friction Model/4(vx [m/s])
  "[y y' x x']"/1 -> Demux1/1
  Ground1/1 -> Mux1/3
  connections:
  F/RConn1 -- Mechanical Branching Bar/LConn1
  Mechanical Branching Bar/RConn1 -- Body Sensor/LConn1
  Mechanical Branching Bar/RConn2 -- Body Actuator/RConn1

== system nms_model/Body Mechanics Layer/Left Heel Contact ==
  note: Planar Ground Interaction Model
  Body Actuator : mblibv1/Sensors &  Actuators/Body Actuator  DialogController=MECH.DynMechDlgSource  SystemSampleTime=-1  UpdateFromCAD=off  PhysicalDomain=Mechanical  PortType=blob  ActuationStyle=Force  AngleUnits=deg  ArcVelocityUnits=deg/s  ArcAccelerationUnits=deg/s^2  CoordPositionUnits=m  VelocityUnits=m/s  AccelerationUnits=m/s^2  ForceUnits=N  TorqueUnits=N-m  ActiveIO=on  Width=3  DialogClass=MechanicalActuatorBlock  ReferenceFrame=Absolute (World)  Angle=off  CoordPosition=on  Force=on  Torque=off
  Body Sensor : mblibv1/Sensors &  Actuators/Body Sensor  DialogController=MECH.DynMechDlgSource  SystemSampleTime=-1  UpdateFromCAD=off  PhysicalDomain=Mechanical  PortType=blob  Muxed=on  Pose=off  Angle=on  AngleUnits=deg  ArcVelocity=off  ArcVelocityUnits=deg/s  ArcAcceleration=off  ArcAccelerationUnits=deg/s^2  CoordPosition=on  CoordPositionUnits=m  Velocity=on  VelocityUnits=m/s  Acceleration=off  AccelerationUnits=m/s^2  Quaternion=on  QuaternionDT=off  QuaternionDDT=off  QuaternionUnits=off  OutputVector=[ 3 3 ]  ActiveIO=on  Width=6  DialogClass=MechanicalSensorBlock  ReferenceFrame=Absolute (World)
  Demux1 : Demux
  Ground Friction Model : Subsystem
  Ground1 : Ground
  Mechanical Branching Bar : mblibv1/Utilities/Mechanical Branching Bar  DialogController=MECH.DynMechDlgSource  PhysicalDomain=mechanical  SubClassName=Unknown  LeftPortType=blob  RightPortType=blob  LConnTagsString=_newl0  RConnTagsString=SA0|SA1  UpdateFromCAD=off  DialogClass=MechanicalBranchingBarBlock  NumSAPorts=2
  Mux : Mux  Inputs=2
  Mux1 : Mux  Inputs=3
  Sum : Sum  Inputs=-+|  OutDataType=sfix(16)  OutScaling=2^0
  Terminator : Terminator
  "[y y' x x']" : Selector  InputPortWidth=6  IndexOptions=Index vector (dialog)  Indices=[2 5 1 4]  OutputSizes=1
  skin contact sensor : simulink/Logic and Bit Operations/Compare To Zero  SystemSampleTime=-1  relop=<=  LogicOutDataTypeMode=boolean
  yGround : Constant  Value=0  OutDataType=fixdt(1, 16)  OutScaling=2^0
  F : PMIOPort  Port=1  Side=Left
  LHeelCnt : Outport  OutDataType=sfix(16)  OutScaling=2^0
  GRF [N N] : Outport  Port=2  OutDataType=sfix(16)  OutScaling=2^0
  wires:
  Ground Friction Model/3(Stiction!) -> Terminator/1
  Ground Friction Model/2(Fx_Friction [N]) -> Mux/1, Mux1/1
  Ground Friction Model/1(Fy_Ground[N]) -> Mux/2, Mux1/2
  skin contact sensor/1 -> Ground Friction Model/Enable, LHeelCnt/1
  Mux/1 -> GRF [N N]/1
  yGround/1 -> Sum/1
  Sum/1 -> Ground Friction Model/1(dy [m]), skin contact sensor/1
  Body Sensor/1 -> "[y y' x x']"/1
  Mux1/1 -> Body Actuator/1
  Demux1/1 -> Sum/2
  Demux1/2 -> Ground Friction Model/2(vy [m/s])
  Demux1/3 -> Ground Friction Model/3(x [m])
  Demux1/4 -> Ground Friction Model/4(vx [m/s])
  "[y y' x x']"/1 -> Demux1/1
  Ground1/1 -> Mux1/3
  connections:
  Mechanical Branching Bar/RConn2 -- Body Actuator/RConn1
  Mechanical Branching Bar/RConn1 -- Body Sensor/LConn1
  F/RConn1 -- Mechanical Branching Bar/LConn1

== system nms_model/Body Mechanics Layer/Left Force Plate ==
  "GRF_Ball [N N] " : Inport  OutDataType=sfix(16)  OutScaling=2^0
  GRF_Heel [N N] : Inport  Port=2  OutDataType=sfix(16)  OutScaling=2^0
  Enable : EnablePort  StatesWhenEnabling=reset
  Fcn : Fcn  Expr=u(1)/(u(2)+eps)
  Mux : Mux  Inputs=3
  Mux1 : Mux  Inputs=2
  Selector : Selector  InputPortWidth=2  IndexOptions=Index vector (dialog)  Indices=2  OutputSizes=1
  Selector1 : Selector  InputPortWidth=2  IndexOptions=Index vector (dialog)  Indices=2  OutputSizes=1
  Sum1 : Sum  OutDataType=sfix(16)  OutScaling=2^0
  GRFs : Outport  OutDataType=sfix(16)  OutScaling=2^0  OutputWhenDisabled=reset  InitialOutput=0
  COP : Outport  Port=2  OutDataType=sfix(16)  OutScaling=2^0  OutputWhenDisabled=reset  InitialOutput=0
  wires:
  Selector/1 -> Mux1/2
  Selector1/1 -> Mux1/1
  "GRF_Ball [N N] "/1 -> Sum1/1, Mux/1, Selector1/1
  GRF_Heel [N N]/1 -> Sum1/2, Mux/3
  Sum1/1 -> Mux/2, Selector/1
  Mux/1 -> GRFs/1
  Mux1/1 -> Fcn/1
  Fcn/1 -> COP/1

== system nms_model/Body Mechanics Layer/Left Thigh Sensor Sheet ==
  note: Inner Segment Pressure Sheet
  Gain3 : Gain  Gain=k_pressure  ParameterDataType=sfix(16)  ParameterScaling=2^0  OutDataType=sfix(16)  OutScaling=2^0
  Gain4 : Gain  Gain=1/v_max_pressure  ParameterDataType=sfix(16)  ParameterScaling=2^0  OutDataType=sfix(16)  OutScaling=2^0
  Inner Thigh Shift Joint : mblibv1/Joints/Prismatic  DialogController=MECH.DynMechDlgSource  PhysicalDomain=mechanical  SubClassName=Unknown  LeftPortType=blob  RightPortType=blob  LConnTagsString=__newl0|SA1|SA2  RConnTagsString=__newr0|SA1  UpdateFromCAD=off  NumSAPorts=3  CutJoint=off  MarkAsCut=off  Primitives=prismatic  PrimitiveProps=P1$WORLD$[1 0 0]$prismatic  DialogClass=JointBlock  P1Axis=[1 0 0]
  Left Thigh Sensor Sheet IC : mblibv1/Sensors &  Actuators/Joint Initial Condition  DialogController=MECH.DynMechDlgSource  SystemSampleTime=-1  UpdateFromCAD=off  PhysicalDomain=mechanical  DialogClass=InitialConditionBlock  InitialConditions=P1$true$0$m$rad$0$m/s$rad/s#P2$false$0$m$rad$0$m/s$rad/s#P3$false$0$m$rad$0$m/s$rad/s#R1$false$0$m$rad$0$m/s$rad/s#R2$false$0$m$rad$0$m/s$rad/s#R3$false$0$m$rad$0$m/s$rad/s#S$false$0$m$rad$0$m/s$rad/s  P1PIC=0  P1VIC=0  P2PIC=0  P2VIC=0  P3PIC=0  P3VIC=0  R1PIC=0  R1VIC=0  R2PIC=0  R2VIC=0  R3PIC=0  R3VIC=0  SPIC=0  SVIC=0
  Mux1 : Mux  Inputs=2
  Pressure Sheet Reaction Force : Fcn  Expr=-u(1) * (1+sgn(u(1))*u(2))
  Thigh Actuator : mblibv1/Sensors &  Actuators/Joint Actuator  DialogController=MECH.DynMechDlgSource  SystemSampleTime=-1  UpdateFromCAD=off  PhysicalDomain=Mechanical  PortType=blob  ActuationStyle=Force  AngleUnits=deg  ArcVelocityUnits=deg/s  ArcAccelerationUnits=deg/s^2  CoordPositionUnits=m  VelocityUnits=m/s  AccelerationUnits=m/s^2  ForceUnits=N  TorqueUnits=N-m  ActiveIO=on  Width=1  DialogClass=MechanicalActuatorBlock  Primitive=P1  ReferenceFrame=Absolute (INERTIAL)
  Thigh Sensor : mblibv1/Sensors &  Actuators/Joint Sensor  DialogController=MECH.DynMechDlgSource  SystemSampleTime=-1  UpdateFromCAD=off  PhysicalDomain=Mechanical  PortType=blob  Muxed=off  Pose=off  Angle=on  AngleUnits=deg  ArcVelocity=off  ArcVelocityUnits=deg/s  ArcAcceleration=off  ArcAccelerationUnits=deg/s^2  CoordPosition=on  CoordPositionUnits=m  Velocity=on  VelocityUnits=m/s  Acceleration=off  AccelerationUnits=m/s^2  Quaternion=on  QuaternionDT=off  QuaternionDDT=off  QuaternionUnits=off  OutputVector=[ 1 1 ]  ActiveIO=on  Width=2  DialogClass=MechanicalSensorBlock  Primitive=P1  Force=off  ForceUnits=N  Torque=off  TorqueUnits=N-m  ReferenceFrame=Absolute (INERTIAL)  ReactionSensedSide=Base  ReactionReferenceFrame=Absolute (World)  ReactionForce=off  ReactionForceUnits=N  ReactionMoment=off  ReactionMomentUnits=N-m
  B : PMIOPort  Tag=PMCPort  Port=1  Side=Left
  F : PMIOPort  Tag=PMCPort  Port=2  Side=Right
  dx : Outport  OutDataType=sfix(16)  OutScaling=2^0
  wires:
  Thigh Sensor/1 -> Gain3/1, dx/1
  Thigh Sensor/2 -> Gain4/1
  Mux1/1 -> Pressure Sheet Reaction Force/1
  Gain3/1 -> Mux1/1
  Gain4/1 -> Mux1/2
  Pressure Sheet Reaction Force/1 -> Thigh Actuator/1
  connections:
  B/RConn1 -- Inner Thigh Shift Joint/LConn1
  F/RConn1 -- Inner Thigh Shift Joint/RConn1
  Thigh Sensor/LConn1 -- Inner Thigh Shift Joint/LConn2
  Inner Thigh Shift Joint/RConn2 -- Thigh Actuator/RConn1
  Left Thigh Sensor Sheet IC/RConn1 -- Inner Thigh Shift Joint/LConn3

== system nms_model/Body Mechanics Layer/Right Ball Contact ==
  note: Planar Ground Interaction Model
  Body Actuator : mblibv1/Sensors &  Actuators/Body Actuator  DialogController=MECH.DynMechDlgSource  SystemSampleTime=-1  UpdateFromCAD=off  PhysicalDomain=Mechanical  PortType=blob  ActuationStyle=Force  AngleUnits=deg  ArcVelocityUnits=deg/s  ArcAccelerationUnits=deg/s^2  CoordPositionUnits=m  VelocityUnits=m/s  AccelerationUnits=m/s^2  ForceUnits=N  TorqueUnits=N-m  ActiveIO=on  Width=3  DialogClass=MechanicalActuatorBlock  ReferenceFrame=Absolute (World)  Angle=off  CoordPosition=on  Force=on  Torque=off
  Body Sensor : mblibv1/Sensors &  Actuators/Body Sensor  DialogController=MECH.DynMechDlgSource  SystemSampleTime=-1  UpdateFromCAD=off  PhysicalDomain=Mechanical  PortType=blob  Muxed=on  Pose=off  Angle=on  AngleUnits=deg  ArcVelocity=off  ArcVelocityUnits=deg/s  ArcAcceleration=off  ArcAccelerationUnits=deg/s^2  CoordPosition=on  CoordPositionUnits=m  Velocity=on  VelocityUnits=m/s  Acceleration=off  AccelerationUnits=m/s^2  Quaternion=on  QuaternionDT=off  QuaternionDDT=off  QuaternionUnits=off  OutputVector=[ 3 3 ]  ActiveIO=on  Width=6  DialogClass=MechanicalSensorBlock  ReferenceFrame=Absolute (World)
  Demux1 : Demux
  Ground : Ground
  Ground Friction Model : Subsystem
  Mechanical Branching Bar : mblibv1/Utilities/Mechanical Branching Bar  DialogController=MECH.DynMechDlgSource  PhysicalDomain=mechanical  SubClassName=Unknown  LeftPortType=blob  RightPortType=blob  LConnTagsString=_newl0  RConnTagsString=SA0|SA1  UpdateFromCAD=off  DialogClass=MechanicalBranchingBarBlock  NumSAPorts=2
  Mux : Mux  Inputs=2
  Mux1 : Mux  Inputs=3
  Sum : Sum  Inputs=-+|  OutDataType=sfix(16)  OutScaling=2^0
  Terminator : Terminator
  "[y y' x x']" : Selector  InputPortWidth=6  IndexOptions=Index vector (dialog)  Indices=[2 5 1 4]  OutputSizes=1
  contact? : simulink/Logic and Bit Operations/Compare To Zero  SystemSampleTime=-1  relop=<=  LogicOutDataTypeMode=boolean
  yGround : Constant  Value=0  OutDataType=fixdt(1, 16)  OutScaling=2^0
  F : PMIOPort  Port=1  Side=Left
  RBallCnt : Outport  OutDataType=sfix(16)  OutScaling=2^0
  GRF [N N] : Outport  Port=2  OutDataType=sfix(16)  OutScaling=2^0
  wires:
  Demux1/2 -> Ground Friction Model/2(vy [m/s])
  contact?/1 -> Ground Friction Model/Enable, RBallCnt/1
  Ground Friction Model/1(Fy_Ground[N]) -> Mux/2, Mux1/2
  Ground Friction Model/2(Fx_Friction [N]) -> Mux/1, Mux1/1
  Ground Friction Model/3(Stiction!) -> Terminator/1
  Mux/1 -> GRF [N N]/1
  Sum/1 -> Ground Friction Model/1(dy [m]), contact?/1
  yGround/1 -> Sum/1
  Body Sensor/1 -> "[y y' x x']"/1
  "[y y' x x']"/1 -> Demux1/1
  Demux1/1 -> Sum/2
  Demux1/3 -> Ground Friction Model/3(x [m])
  Demux1/4 -> Ground Friction Model/4(vx [m/s])
  Ground/1 -> Mux1/3
  Mux1/1 -> Body Actuator/1
  connections:
  F/RConn1 -- Mechanical Branching Bar/LConn1
  Mechanical Branching Bar/RConn2 -- Body Actuator/RConn1
  Mechanical Branching Bar/RConn1 -- Body Sensor/LConn1

== system nms_model/Body Mechanics Layer/Right Heel Contact ==
  note: Planar Ground Interaction Model
  Body Actuator : mblibv1/Sensors &  Actuators/Body Actuator  DialogController=MECH.DynMechDlgSource  SystemSampleTime=-1  UpdateFromCAD=off  PhysicalDomain=Mechanical  PortType=blob  ActuationStyle=Force  AngleUnits=deg  ArcVelocityUnits=deg/s  ArcAccelerationUnits=deg/s^2  CoordPositionUnits=m  VelocityUnits=m/s  AccelerationUnits=m/s^2  ForceUnits=N  TorqueUnits=N-m  ActiveIO=on  Width=3  DialogClass=MechanicalActuatorBlock  ReferenceFrame=Absolute (World)  Angle=off  CoordPosition=on  Force=on  Torque=off
  Body Sensor : mblibv1/Sensors &  Actuators/Body Sensor  DialogController=MECH.DynMechDlgSource  SystemSampleTime=-1  UpdateFromCAD=off  PhysicalDomain=Mechanical  PortType=blob  Muxed=on  Pose=off  Angle=on  AngleUnits=deg  ArcVelocity=off  ArcVelocityUnits=deg/s  ArcAcceleration=off  ArcAccelerationUnits=deg/s^2  CoordPosition=on  CoordPositionUnits=m  Velocity=on  VelocityUnits=m/s  Acceleration=off  AccelerationUnits=m/s^2  Quaternion=on  QuaternionDT=off  QuaternionDDT=off  QuaternionUnits=off  OutputVector=[ 3 3 ]  ActiveIO=on  Width=6  DialogClass=MechanicalSensorBlock  ReferenceFrame=Absolute (World)
  Demux1 : Demux
  Ground : Ground
  Ground Friction Model : Subsystem
  Mechanical Branching Bar : mblibv1/Utilities/Mechanical Branching Bar  DialogController=MECH.DynMechDlgSource  PhysicalDomain=mechanical  SubClassName=Unknown  LeftPortType=blob  RightPortType=blob  LConnTagsString=_newl0  RConnTagsString=SA0|SA1  UpdateFromCAD=off  DialogClass=MechanicalBranchingBarBlock  NumSAPorts=2
  Mux : Mux  Inputs=2
  Mux1 : Mux  Inputs=3
  Sum : Sum  Inputs=-+|  OutDataType=sfix(16)  OutScaling=2^0
  Terminator : Terminator
  "[y y' x x']" : Selector  InputPortWidth=6  IndexOptions=Index vector (dialog)  Indices=[2 5 1 4]  OutputSizes=1
  contact? : simulink/Logic and Bit Operations/Compare To Zero  SystemSampleTime=-1  relop=<=  LogicOutDataTypeMode=boolean
  yGround : Constant  Value=0  OutDataType=fixdt(1, 16)  OutScaling=2^0
  F : PMIOPort  Port=1  Side=Left
  RHeelCnt : Outport  OutDataType=sfix(16)  OutScaling=2^0
  GRF [N N] : Outport  Port=2  OutDataType=sfix(16)  OutScaling=2^0
  wires:
  Ground Friction Model/3(Stiction!) -> Terminator/1
  Ground Friction Model/2(Fx_Friction [N]) -> Mux/1, Mux1/1
  Ground Friction Model/1(Fy_Ground[N]) -> Mux/2, Mux1/2
  contact?/1 -> Ground Friction Model/Enable, RHeelCnt/1
  Demux1/4 -> Ground Friction Model/4(vx [m/s])
  Demux1/3 -> Ground Friction Model/3(x [m])
  Demux1/2 -> Ground Friction Model/2(vy [m/s])
  Mux/1 -> GRF [N N]/1
  yGround/1 -> Sum/1
  Demux1/1 -> Sum/2  "yBall"
  Sum/1 -> Ground Friction Model/1(dy [m]), contact?/1
  Body Sensor/1 -> "[y y' x x']"/1
  "[y y' x x']"/1 -> Demux1/1
  Mux1/1 -> Body Actuator/1
  Ground/1 -> Mux1/3
  connections:
  F/RConn1 -- Mechanical Branching Bar/LConn1
  Mechanical Branching Bar/RConn1 -- Body Sensor/LConn1
  Mechanical Branching Bar/RConn2 -- Body Actuator/RConn1

== system nms_model/Body Mechanics Layer/Right Force Plate ==
  "GRF_Ball [N N] " : Inport  OutDataType=sfix(16)  OutScaling=2^0
  GRF_Heel [N N] : Inport  Port=2  OutDataType=sfix(16)  OutScaling=2^0
  Enable : EnablePort  StatesWhenEnabling=reset
  Fcn : Fcn  Expr=u(1)/(u(2)+eps)
  Mux : Mux  Inputs=3
  Mux1 : Mux  Inputs=2
  Selector : Selector  InputPortWidth=2  IndexOptions=Index vector (dialog)  Indices=2  OutputSizes=1
  Selector1 : Selector  InputPortWidth=2  IndexOptions=Index vector (dialog)  Indices=2  OutputSizes=1
  Sum1 : Sum  OutDataType=sfix(16)  OutScaling=2^0
  GRFs : Outport  OutDataType=sfix(16)  OutScaling=2^0  OutputWhenDisabled=reset  InitialOutput=0
  COP : Outport  Port=2  OutDataType=sfix(16)  OutScaling=2^0  OutputWhenDisabled=reset  InitialOutput=0
  wires:
  Selector/1 -> Mux1/2
  Selector1/1 -> Mux1/1
  "GRF_Ball [N N] "/1 -> Sum1/1, Mux/1, Selector1/1
  GRF_Heel [N N]/1 -> Sum1/2, Mux/3
  Sum1/1 -> Mux/2, Selector/1
  Mux/1 -> GRFs/1
  Mux1/1 -> Fcn/1
  Fcn/1 -> COP/1
